simulink model "qbdelta_r2018"  (R2018a)
settings: Solver=ode1  StartTime=0.0  StopTime=20  FixedStep=0.005  RelTol=1e-3
InitFcn:
  | delta = delta_init('qbdelta');
libraries: qbmove_library x2
settings Model: EnablePacing=on  Creator=alextoind  LastModifiedBy=alextoind
settings HardwareCC: ProdBitPerLong=64  ProdHWDeviceType=Intel->x86-64 (Linux 64)
settings SFSimCC: SimUseLocalCustomCode=on
settings RTWCC: RTWUseLocalCustomCode=on
settings CodeAppCC: StateflowObjectComments=on

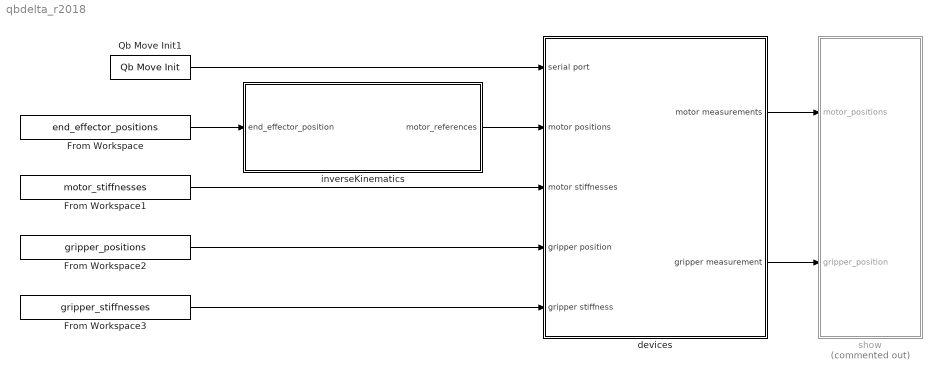
== system qbdelta_r2018 ==
  From Workspace : FromWorkspace  VariableName=end_effector_positions  SampleTime=0
  From Workspace1 : FromWorkspace  VariableName=motor_stiffnesses  SampleTime=0
  From Workspace2 : FromWorkspace  VariableName=gripper_positions  SampleTime=0
  From Workspace3 : FromWorkspace  VariableName=gripper_stiffnesses  SampleTime=0
  Qb Move Init1 : qbmove_library/Qb Move Init  NUMBER_OF_COM='/dev/ttyUSB1'  BAUD_RATE_COM=2000000
      settings: SourceProductName=Qb Move Library
  devices : Subsystem
  inverseKinematics : MATLAB Function  TreatAsAtomicUnit=on
  show : MATLAB Function  Commented=on  TreatAsAtomicUnit=on
  wires:
  Qb Move Init1/1 -> devices/1(serial port)
  From Workspace2/1 -> devices/4(gripper position)
  From Workspace3/1 -> devices/5(gripper stiffness)
  From Workspace1/1 -> devices/3(motor stiffnesses)
  From Workspace/1 -> inverseKinematics/1(end_effector_position)
  devices/1(motor measurements) -> show/1(motor_positions)
  inverseKinematics/1(motor_references) -> devices/2(motor positions)
  devices/2(gripper measurement) -> show/2(gripper_position)

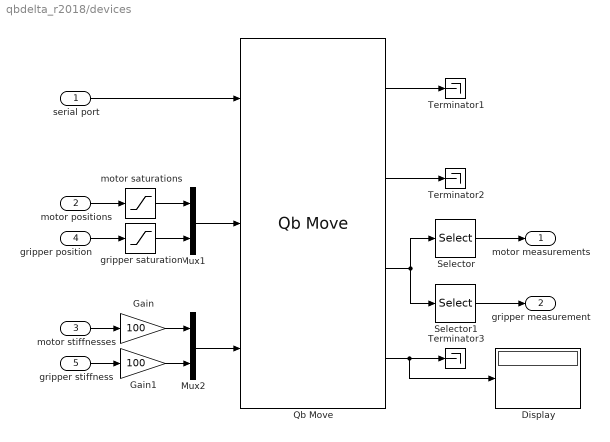
== system qbdelta_r2018/devices ==
  serial port : Inport
  motor positions : Inport  Port=2
  motor stiffnesses : Inport  Port=3
  gripper position : Inport  Port=4
  gripper stiffness : Inport  Port=5
  Display : Display
  Gain : Gain  Gain=100
  Gain1 : Gain  Gain=100
  Mux1 : Mux  Inputs=2
  Mux2 : Mux  Inputs=2
  Qb Move : qbmove_library/Qb Move  ID=[1 2 3 4]  ACTIVE_COMM_DIRECTIONS=Both  CONTROL_MODE=Equilibrium Position and Stiffness Preset Percentage  DAISY_CHAINING=off  MAX_ANG=0  SW_LIMIT=inf  OFFSET=0  ACTIVATE=on  WDT=0.0  UNIT=Radians  INPUTS_ACK=off
      settings: SourceProductName=Qb Move Library
  Selector : Selector  InputPortWidth=4  IndexOptions=Index vector (dialog)  Indices=[1 2 3]  OutputSizes=1
  Selector1 : Selector  InputPortWidth=4  IndexOptions=Index vector (dialog)  Indices=[4]  OutputSizes=1
  Terminator1 : Terminator
  Terminator2 : Terminator
  Terminator3 : Terminator
  gripper saturation : Saturate  UpperLimit=1.4  LowerLimit=0
  motor saturations : Saturate  UpperLimit=1.0  LowerLimit=-1.5
  motor measurements : Outport
  gripper measurement : Outport  Port=2
  wires:
  motor positions/1 -> motor saturations/1
  Qb Move/1 -> Terminator1/1
  Qb Move/2 -> Terminator2/1
  Qb Move/4 -> Display/1, Terminator3/1
  serial port/1 -> Qb Move/1
  motor saturations/1 -> Mux1/1
  Mux2/1 -> Qb Move/3
  Mux1/1 -> Qb Move/2
  gripper position/1 -> gripper saturation/1
  gripper stiffness/1 -> Gain1/1
  motor stiffnesses/1 -> Gain/1
  Qb Move/3 -> Selector/1, Selector1/1
  Selector/1 -> motor measurements/1
  gripper saturation/1 -> Mux1/2
  Gain/1 -> Mux2/1
  Gain1/1 -> Mux2/2
  Selector1/1 -> gripper measurement/1

== matlab function qbdelta_r2018/show ==
  data: motor_positions input; gripper_position input
function show(motor_positions, gripper_position)
  coder.extrinsic('delta_show');
  coder.extrinsic('evalin')

  delta = evalin('base', 'delta');
  delta_show(delta, motor_positions, gripper_position);
end

== matlab function qbdelta_r2018/inverseKinematics ==
  settings: updateMethod=DISCRETE
  data: end_effector_position input; motor_references output
function motor_references = inverseKinematics(end_effector_position)
  coder.extrinsic('delta_ik');

  persistent last_motor_references_;
  if isempty(last_motor_references_)
    last_motor_references_ = zeros(3,1);
  end

  motor_references = zeros(3,1);  % Simulink needs to know the size because of extrinsic function
  [isvalid, motor_references] = delta_ik(end_effector_position);
  if ~isvalid
    motor_references = last_motor_references_;
    return;
  end
  last_motor_references_ = motor_references;
end
